simulink model "benchmark_LT"  (Simulink 7.0)
settings: Solver=ode45  SolverMode=SingleTasking  StartTime=0.0  StopTime=609  FixedStep=0.01  RelTol=1e-5  AbsTol=1e-8
values from neighbouring files (symbols this model uses):
  ACTIVATE = [0]    [benchmarkinit.m]
  DECAY = [0]    [benchmarkinit.m]
  TEMPMODEL = [0]    [benchmarkinit.m]
undefined symbols (not defined in the file or in its folder): carb1, carb2, carb3, carb4, carb5, KLa1, KLa2, KLa3, KLa4, KLa5, PAR1, PAR2, PAR3, PAR4, PAR5, Qin0, Qintr, Qw, SOSAT2, SOSAT3, SOSAT4, SOSAT5, T, VOL2, VOL3, VOL4, VOL5, XINIT, XINIT2, XINIT3, XINIT4, XINIT5
settings Model: Creator=ielulf  LastModifiedBy=xavier  ExtModeTrigMode=oneshot  ExtModeArmWhenConnect=off  ExtModeAutoUpdateStatusClock=off
settings DataIOCC: LimitDataPoints=off  SaveOutput=off  TimeSaveName=t  SignalLoggingName=sigsOut  OutputOption=SpecifiedOutputTimes  OutputTimes=[245:(1/96):609]
settings OptimizationCC: BlockReduction=off  BooleanDataType=off
settings DebuggingCC: AlgebraicLoopMsg=none  SaveWithParameterizedLinksMsg=none  SignalResolutionControl=TryResolveAllWithWarning  SolverPrmCheckMsg=none  InheritedTsInSrcMsg=none  MultiTaskDSMMsg=warning  MultiTaskCondExecSysMsg=none  UnconnectedOutputMsg=none  StrictBusMsg=None
settings HardwareCC: TargetUnknown=on
settings RTWCC: TemplateMakefile=grt_unix.tmf  IncludeERTFirstTime=on
settings GRTTargetCC: TargetFcnLib=ansi_tfl_tmw.mat

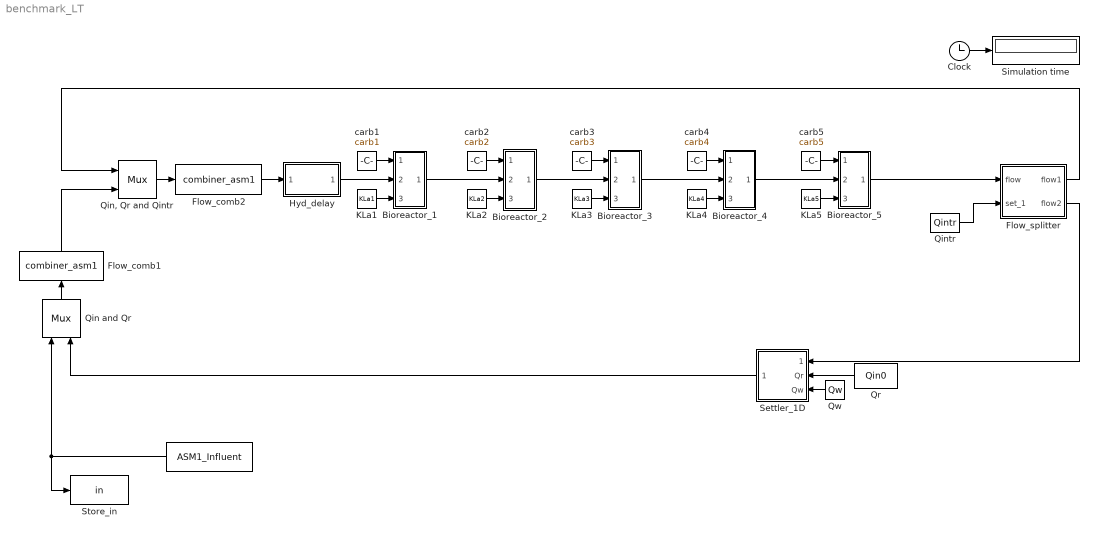
== system benchmark_LT ==
  " " : FromWorkspace  Orientation=left  VariableName=ASM1_Influent  OutputAfterFinalValue=Holding final value
  Bioreactor_1 : Subsystem
  Bioreactor_2 : Subsystem
  Bioreactor_3 : Subsystem
  Bioreactor_4 : Subsystem
  Bioreactor_5 : Subsystem
  Clock : Clock
      settings: Decimation=10
  Flow_comb1 : S-Function  Orientation=up  FunctionName=combiner_asm1
  Flow_comb2 : S-Function  FunctionName=combiner_asm1
  Flow_splitter : Subsystem
  Hyd_delay : Subsystem
  KLa1 : Constant  Value=KLa1  OutDataType=sfix(16)  OutScaling=2^0
  KLa2 : Constant  Value=KLa2  OutDataType=sfix(16)  OutScaling=2^0
  KLa3 : Constant  Value=KLa3  OutDataType=sfix(16)  OutScaling=2^0
  KLa4 : Constant  Value=KLa4  OutDataType=sfix(16)  OutScaling=2^0
  KLa5 : Constant  Value=KLa5  OutDataType=sfix(16)  OutScaling=2^0
  Qin and Qr : Mux  Orientation=up  Inputs=2
  "Qin, Qr and Qintr" : Mux  Inputs=2
  Qintr : Constant  Value=Qintr  OutDataType=sfix(16)  OutScaling=2^0
  Qr : Constant  Orientation=left  Value=Qin0  OutDataType=sfix(16)  OutScaling=2^0
  Qw : Constant  Orientation=left  Value=Qw  OutDataType=sfix(16)  OutScaling=2^0
  Settler_1D : Subsystem  Orientation=left
  Simulation time : Display
  Store_in : ToWorkspace  VariableName=in  SampleTime=-1  SaveFormat=Array
  carb1 : Constant  Value=carb1  OutDataType=sfix(16)  OutScaling=2^0
  carb2 : Constant  Value=carb2  OutDataType=sfix(16)  OutScaling=2^0
  carb3 : Constant  Value=carb3  OutDataType=sfix(16)  OutScaling=2^0
  carb4 : Constant  Value=carb4  OutDataType=sfix(16)  OutScaling=2^0
  carb5 : Constant  Value=carb5  OutDataType=sfix(16)  OutScaling=2^0
  wires:
  Qin and Qr/1 -> Flow_comb1/1
  Flow_comb1/1 -> "Qin, Qr and Qintr"/2
  "Qin, Qr and Qintr"/1 -> Flow_comb2/1
  Flow_splitter/1(flow1) -> "Qin, Qr and Qintr"/1
  Settler_1D/1(output) -> Qin and Qr/2
  Qw/1 -> Settler_1D/3(Qw)
  Flow_splitter/2(flow2) -> Settler_1D/1(feed)
  Qr/1 -> Settler_1D/2(Qr)
  Bioreactor_5/1(out) -> Flow_splitter/1(flow)
  Flow_comb2/1 -> Hyd_delay/1(Input)
  Clock/1 -> Simulation time/1
  Hyd_delay/1(Output) -> Bioreactor_1/2(in)
  carb1/1 -> Bioreactor_1/1(carb)
  KLa1/1 -> Bioreactor_1/3(KLa)
  Bioreactor_1/1(out) -> Bioreactor_2/2(in)
  KLa2/1 -> Bioreactor_2/3(KLa)
  carb2/1 -> Bioreactor_2/1(carb)
  Bioreactor_2/1(out) -> Bioreactor_3/2(in)
  KLa3/1 -> Bioreactor_3/3(KLa)
  carb3/1 -> Bioreactor_3/1(carb)
  Bioreactor_3/1(out) -> Bioreactor_4/2(in)
  KLa4/1 -> Bioreactor_4/3(KLa)
  carb4/1 -> Bioreactor_4/1(carb)
  Bioreactor_4/1(out) -> Bioreactor_5/2(in)
  carb5/1 -> Bioreactor_5/1(carb)
  " "/1 -> Store_in/1, Qin and Qr/1
  KLa5/1 -> Bioreactor_5/3(KLa)
  Qintr/1 -> Flow_splitter/2(set_1)

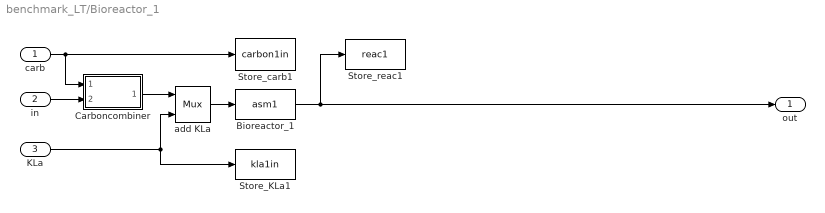
== system benchmark_LT/Bioreactor_1 ==
  carb : Inport  OutDataType=sfix(16)  OutScaling=2^0
  in : Inport  Port=2  OutDataType=sfix(16)  OutScaling=2^0
  KLa : Inport  Port=3  OutDataType=sfix(16)  OutScaling=2^0
  Bioreactor_1 : S-Function  FunctionName=asm1  Parameters=XINIT1,PAR1,VOL1,SOSAT1, TEMPMODEL,ACTIVATE, DECAY
  Carboncombiner : Subsystem
  Store_KLa1 : ToWorkspace  VariableName=kla1in  SampleTime=-1  SaveFormat=Array
  Store_carb1 : ToWorkspace  VariableName=carbon1in  SampleTime=-1  SaveFormat=Array
  Store_reac1 : ToWorkspace  VariableName=reac1  SampleTime=-1  SaveFormat=Array
  add KLa : Mux  Inputs=2
  out : Outport  OutDataType=sfix(16)  OutScaling=2^0
  wires:
  add KLa/1 -> Bioreactor_1/1
  Bioreactor_1/1 -> Store_reac1/1, out/1
  Carboncombiner/1(Output) -> add KLa/1
  carb/1 -> Store_carb1/1, Carboncombiner/1(C_flow)
  in/1 -> Carboncombiner/2(Input)
  KLa/1 -> add KLa/2, Store_KLa1/1

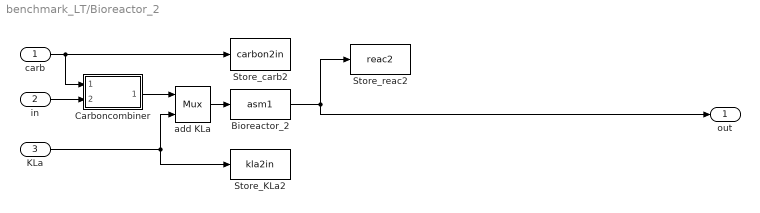
== system benchmark_LT/Bioreactor_2 ==
  carb : Inport  OutDataType=sfix(16)  OutScaling=2^0
  in : Inport  Port=2  OutDataType=sfix(16)  OutScaling=2^0
  KLa : Inport  Port=3  OutDataType=sfix(16)  OutScaling=2^0
  Bioreactor_2 : S-Function  FunctionName=asm1  Parameters=XINIT2,PAR2,VOL2,SOSAT2,TEMPMODEL,ACTIVATE,DECAY
  Carboncombiner : Subsystem
  Store_KLa2 : ToWorkspace  VariableName=kla2in  SampleTime=-1  SaveFormat=Array
  Store_carb2 : ToWorkspace  VariableName=carbon2in  SampleTime=-1  SaveFormat=Array
  Store_reac2 : ToWorkspace  VariableName=reac2  SampleTime=-1  SaveFormat=Array
  add KLa : Mux  Inputs=2
  out : Outport  OutDataType=sfix(16)  OutScaling=2^0
  wires:
  Bioreactor_2/1 -> Store_reac2/1, out/1
  add KLa/1 -> Bioreactor_2/1
  Carboncombiner/1(Output) -> add KLa/1
  carb/1 -> Carboncombiner/1(C_flow), Store_carb2/1
  in/1 -> Carboncombiner/2(Input)
  KLa/1 -> add KLa/2, Store_KLa2/1

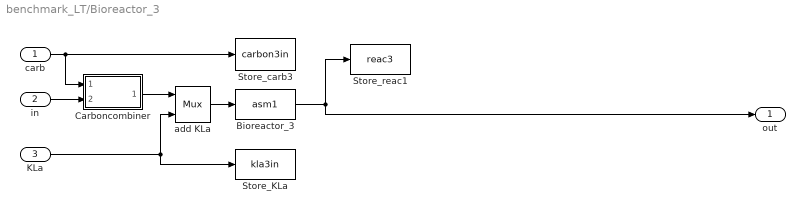
== system benchmark_LT/Bioreactor_3 ==
  carb : Inport  OutDataType=sfix(16)  OutScaling=2^0
  in : Inport  Port=2  OutDataType=sfix(16)  OutScaling=2^0
  KLa : Inport  Port=3  OutDataType=sfix(16)  OutScaling=2^0
  Bioreactor_3 : S-Function  FunctionName=asm1  Parameters=XINIT3,PAR3,VOL3,SOSAT3,TEMPMODEL,ACTIVATE,DECAY
  Carboncombiner : Subsystem
  Store_KLa : ToWorkspace  VariableName=kla3in  SampleTime=-1  SaveFormat=Array
  Store_carb3 : ToWorkspace  VariableName=carbon3in  SampleTime=-1  SaveFormat=Array
  Store_reac1 : ToWorkspace  VariableName=reac3  SampleTime=-1  SaveFormat=Array
  add KLa : Mux  Inputs=2
  out : Outport  OutDataType=sfix(16)  OutScaling=2^0
  wires:
  Bioreactor_3/1 -> Store_reac1/1, out/1
  add KLa/1 -> Bioreactor_3/1
  Carboncombiner/1(Output) -> add KLa/1
  carb/1 -> Carboncombiner/1(C_flow), Store_carb3/1
  in/1 -> Carboncombiner/2(Input)
  KLa/1 -> add KLa/2, Store_KLa/1

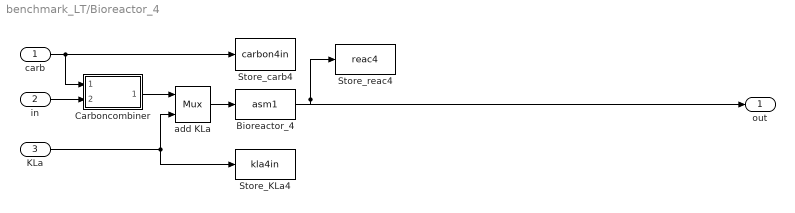
== system benchmark_LT/Bioreactor_4 ==
  carb : Inport  OutDataType=sfix(16)  OutScaling=2^0
  in : Inport  Port=2  OutDataType=sfix(16)  OutScaling=2^0
  KLa : Inport  Port=3  OutDataType=sfix(16)  OutScaling=2^0
  Bioreactor_4 : S-Function  FunctionName=asm1  Parameters=XINIT4,PAR4,VOL4,SOSAT4,TEMPMODEL,ACTIVATE,DECAY
  Carboncombiner : Subsystem
  Store_KLa4 : ToWorkspace  VariableName=kla4in  SampleTime=-1  SaveFormat=Array
  Store_carb4 : ToWorkspace  VariableName=carbon4in  SampleTime=-1  SaveFormat=Array
  Store_reac4 : ToWorkspace  VariableName=reac4  SampleTime=-1  SaveFormat=Array
  add KLa : Mux  Inputs=2
  out : Outport  OutDataType=sfix(16)  OutScaling=2^0
  wires:
  Bioreactor_4/1 -> Store_reac4/1, out/1
  add KLa/1 -> Bioreactor_4/1
  Carboncombiner/1(Output) -> add KLa/1
  carb/1 -> Carboncombiner/1(C_flow), Store_carb4/1
  in/1 -> Carboncombiner/2(Input)
  KLa/1 -> add KLa/2, Store_KLa4/1

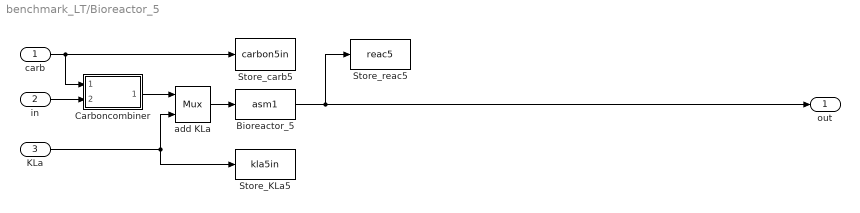
== system benchmark_LT/Bioreactor_5 ==
  carb : Inport  OutDataType=sfix(16)  OutScaling=2^0
  in : Inport  Port=2  OutDataType=sfix(16)  OutScaling=2^0
  KLa : Inport  Port=3  OutDataType=sfix(16)  OutScaling=2^0
  Bioreactor_5 : S-Function  FunctionName=asm1  Parameters=XINIT5,PAR5,VOL5,SOSAT5,TEMPMODEL,ACTIVATE,DECAY
  Carboncombiner : Subsystem
  Store_KLa5 : ToWorkspace  VariableName=kla5in  SampleTime=-1  SaveFormat=Array
  Store_carb5 : ToWorkspace  VariableName=carbon5in  SampleTime=-1  SaveFormat=Array
  Store_reac5 : ToWorkspace  VariableName=reac5  SampleTime=-1  SaveFormat=Array
  add KLa : Mux  Inputs=2
  out : Outport  OutDataType=sfix(16)  OutScaling=2^0
  wires:
  Bioreactor_5/1 -> Store_reac5/1, out/1
  add KLa/1 -> Bioreactor_5/1
  Carboncombiner/1(Output) -> add KLa/1
  carb/1 -> Carboncombiner/1(C_flow), Store_carb5/1
  in/1 -> Carboncombiner/2(Input)
  KLa/1 -> add KLa/2, Store_KLa5/1

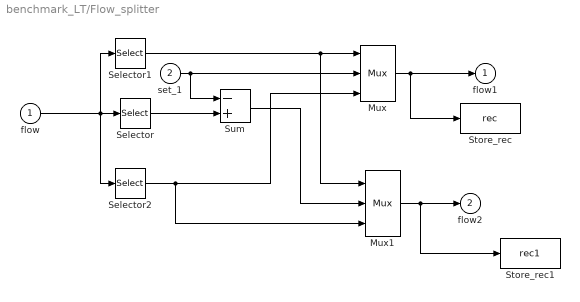
== system benchmark_LT/Flow_splitter ==
  flow : Inport  OutDataType=sfix(16)  OutScaling=2^0
  set_1 : Inport  Port=2  OutDataType=sfix(16)  OutScaling=2^0
  Mux : Mux  Inputs=3
  Mux1 : Mux  Inputs=3
  Selector : Selector  InputPortWidth=21  IndexOptions=Index vector (dialog)  Indices=[15]  OutputSizes=1
  Selector1 : Selector  InputPortWidth=21  IndexOptions=Index vector (dialog)  Indices=[1 2 3 4 5 6 7 8 9 10 11 12 13 14]  OutputSizes=1
  Selector2 : Selector  InputPortWidth=21  IndexOptions=Index vector (dialog)  Indices=[16 17 18 19 20 21]  OutputSizes=1
  Store_rec : ToWorkspace  VariableName=rec  SampleTime=-1  SaveFormat=Array
  Store_rec1 : ToWorkspace  VariableName=rec1  SampleTime=-1  SaveFormat=Array
  Sum : Sum  Inputs=-+  OutDataType=sfix(16)  OutScaling=2^0  SaturateOnIntegerOverflow=on  InputSameDT=on
  flow1 : Outport  OutDataType=sfix(16)  OutScaling=2^0
  flow2 : Outport  Port=2  OutDataType=sfix(16)  OutScaling=2^0
  wires:
  flow/1 -> Selector1/1, Selector/1, Selector2/1
  Mux/1 -> flow1/1, Store_rec/1
  Mux1/1 -> flow2/1, Store_rec1/1
  set_1/1 -> Mux/2, Sum/1
  Selector/1 -> Sum/2
  Sum/1 -> Mux1/2
  Selector1/1 -> Mux/1, Mux1/1
  Selector2/1 -> Mux/3, Mux1/3

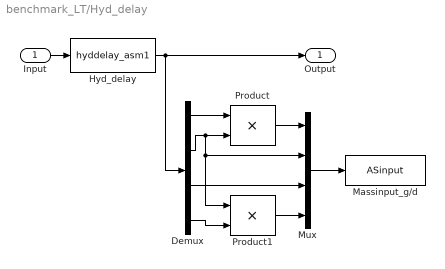
== system benchmark_LT/Hyd_delay ==
  Input : Inport  OutDataType=sfix(16)  OutScaling=2^0
  Demux : Demux  Outputs=[14,1,1,5]
  Hyd_delay : S-Function  FunctionName=hyddelay_asm1  Parameters=XINIT,PAR1,T
  Massinput_g/d : ToWorkspace  VariableName=ASinput  SampleTime=-1  SaveFormat=Array
  Mux : Mux
  Product : Product  OutDataType=sfix(16)  OutScaling=2^0  SaturateOnIntegerOverflow=on
  Product1 : Product  OutDataType=sfix(16)  OutScaling=2^0  SaturateOnIntegerOverflow=on
  Output : Outport  OutDataType=sfix(16)  OutScaling=2^0
  wires:
  Demux/4 -> Product1/2
  Product1/1 -> Mux/4
  Demux/3 -> Mux/3
  Demux/2 -> Product1/1, Mux/2, Product/2
  Input/1 -> Hyd_delay/1
  Hyd_delay/1 -> Demux/1, Output/1
  Demux/1 -> Product/1
  Product/1 -> Mux/1
  Mux/1 -> Massinput_g/d/1

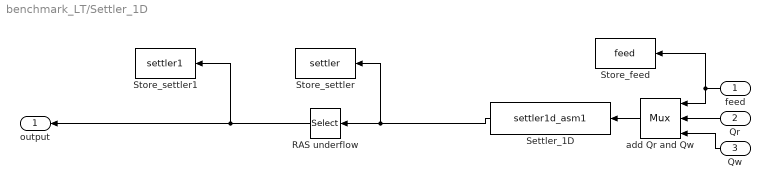
== system benchmark_LT/Settler_1D ==
  feed : Inport  Orientation=left  OutDataType=sfix(16)  OutScaling=2^0
  Qr : Inport  Orientation=left  Port=2  OutDataType=sfix(16)  OutScaling=2^0
  Qw : Inport  Orientation=left  Port=3  OutDataType=sfix(16)  OutScaling=2^0
  RAS underflow : Selector  Orientation=left  InputPortWidth=203  IndexOptions=Index vector (dialog)  Indices=[181 182 183 184 185 186 187 188 189 190 191 192 193 194 202 195 196 197 198 199 200]  OutputSizes=1
  Settler_1D : S-Function  Orientation=left  FunctionName=settler1d_asm1  Parameters=SETTLERINIT,SETTLERPAR,DIM,LAYER,PAR1,TEMPMODEL, DECAY, SETTLER
  Store_feed : ToWorkspace  VariableName=feed  SampleTime=-1  SaveFormat=Array
  Store_settler : ToWorkspace  VariableName=settler  SampleTime=-1  SaveFormat=Array
  Store_settler1 : ToWorkspace  VariableName=settler1  SampleTime=-1  SaveFormat=Array
  add Qr and Qw : Mux  Orientation=left  Inputs=3
  output : Outport  Orientation=left  OutDataType=sfix(16)  OutScaling=2^0
  wires:
  add Qr and Qw/1 -> Settler_1D/1
  Qr/1 -> add Qr and Qw/2
  Qw/1 -> add Qr and Qw/3
  feed/1 -> add Qr and Qw/1, Store_feed/1
  RAS underflow/1 -> output/1, Store_settler1/1
  Settler_1D/1 -> RAS underflow/1, Store_settler/1

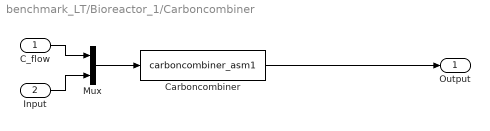
== system benchmark_LT/Bioreactor_1/Carboncombiner ==
  C_flow : Inport  OutDataType=sfix(16)  OutScaling=2^0
  Input : Inport  Port=2  OutDataType=sfix(16)  OutScaling=2^0
  Carboncombiner : S-Function  FunctionName=carboncombiner_asm1  Parameters=CARBONSOURCECONC
  Mux : Mux  Inputs=2
  Output : Outport  OutDataType=sfix(16)  OutScaling=2^0
  wires:
  C_flow/1 -> Mux/1
  Mux/1 -> Carboncombiner/1
  Carboncombiner/1 -> Output/1
  Input/1 -> Mux/2

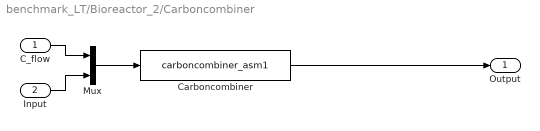
== system benchmark_LT/Bioreactor_2/Carboncombiner ==
  C_flow : Inport  OutDataType=sfix(16)  OutScaling=2^0
  Input : Inport  Port=2  OutDataType=sfix(16)  OutScaling=2^0
  Carboncombiner : S-Function  FunctionName=carboncombiner_asm1  Parameters=CARBONSOURCECONC
  Mux : Mux  Inputs=2
  Output : Outport  OutDataType=sfix(16)  OutScaling=2^0
  wires:
  Input/1 -> Mux/2
  Carboncombiner/1 -> Output/1
  Mux/1 -> Carboncombiner/1
  C_flow/1 -> Mux/1

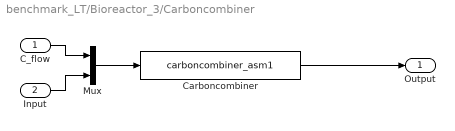
== system benchmark_LT/Bioreactor_3/Carboncombiner ==
  C_flow : Inport  OutDataType=sfix(16)  OutScaling=2^0
  Input : Inport  Port=2  OutDataType=sfix(16)  OutScaling=2^0
  Carboncombiner : S-Function  FunctionName=carboncombiner_asm1  Parameters=CARBONSOURCECONC
  Mux : Mux  Inputs=2
  Output : Outport  OutDataType=sfix(16)  OutScaling=2^0
  wires:
  Input/1 -> Mux/2
  Carboncombiner/1 -> Output/1
  Mux/1 -> Carboncombiner/1
  C_flow/1 -> Mux/1

== system benchmark_LT/Bioreactor_4/Carboncombiner ==
  C_flow : Inport  OutDataType=sfix(16)  OutScaling=2^0
  Input : Inport  Port=2  OutDataType=sfix(16)  OutScaling=2^0
  Carboncombiner : S-Function  FunctionName=carboncombiner_asm1  Parameters=CARBONSOURCECONC
  Mux : Mux  Inputs=2
  Output : Outport  OutDataType=sfix(16)  OutScaling=2^0
  wires:
  Input/1 -> Mux/2
  Carboncombiner/1 -> Output/1
  Mux/1 -> Carboncombiner/1
  C_flow/1 -> Mux/1

== system benchmark_LT/Bioreactor_5/Carboncombiner ==
  C_flow : Inport  OutDataType=sfix(16)  OutScaling=2^0
  Input : Inport  Port=2  OutDataType=sfix(16)  OutScaling=2^0
  Carboncombiner : S-Function  FunctionName=carboncombiner_asm1  Parameters=CARBONSOURCECONC
  Mux : Mux  Inputs=2
  Output : Outport  OutDataType=sfix(16)  OutScaling=2^0
  wires:
  Input/1 -> Mux/2
  Carboncombiner/1 -> Output/1
  Mux/1 -> Carboncombiner/1
  C_flow/1 -> Mux/1
